simulink subsystem "Ultrasonic_Motor_Head"  (R2020b)
settings: Solver=VariableStepAuto  StartTime=0.0  StopTime=10.0  RelTol=1e-3
libraries: simulink_extras x1
settings Model: Creator=rthom  LastModifiedBy=david

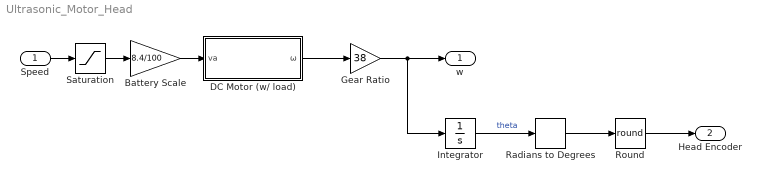
== system Ultrasonic_Motor_Head ==
  Speed : Inport
  Battery Scale : Gain  Gain=8.4/100
  DC Motor (w/ load) : Subsystem
  Gear Ratio : Gain  Gain=38
  Integrator : Integrator
  Radians to Degrees : simulink_extras/Transformations/Radians to Degrees
  Round : Rounding  Operator=round
  Saturation : Saturate  UpperLimit=100  LowerLimit=-100
  w : Outport
  Head Encoder : Outport  Port=2
  wires:
  Battery Scale/1 -> DC Motor (w/ load)/1(va)
  Round/1 -> Head Encoder/1
  Radians to Degrees/1 -> Round/1
  Integrator/1 -> Radians to Degrees/1  "theta"
  Saturation/1 -> Battery Scale/1
  Speed/1 -> Saturation/1
  Gear Ratio/1 -> Integrator/1, w/1
  DC Motor (w/ load)/1(ω) -> Gear Ratio/1

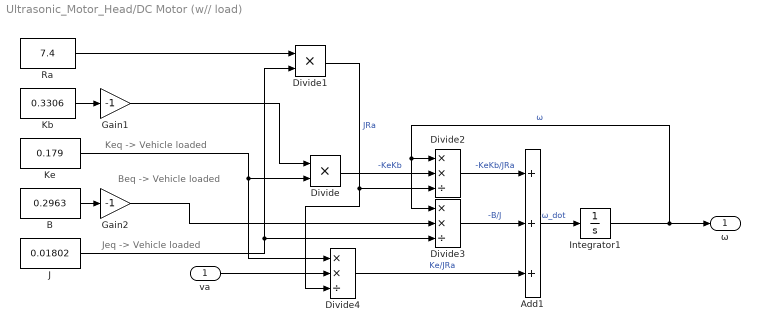
== system Ultrasonic_Motor_Head/DC Motor (w// load) ==
  note: Keq -> Vehicle loaded
  note: Jeq -> Vehicle loaded
  note: Beq -> Vehicle loaded
  va : Inport
  Add1 : Sum  Inputs=+++
  B : Constant  Value=0.2963
  Divide : Product  Inputs=**
  Divide1 : Product  Inputs=**
  Divide2 : Product  Inputs=**/
  Divide3 : Product  Inputs=**/
  Divide4 : Product  Inputs=**/
  Gain1 : Gain  Gain=-1
  Gain2 : Gain  Gain=-1
  Integrator1 : Integrator
  J : Constant  Value=0.01802
  Kb : Constant  Value=0.3306
  Ke : Constant  Value=0.179
  Ra : Constant  Value=7.4
  ω : Outport
  wires:
  Divide3/1 -> Add1/2  "-B/J"
  Add1/1 -> Integrator1/1  "ω_dot"
  J/1 -> Divide3/3, Divide1/2
  va/1 -> Divide4/2
  Ke/1 -> Divide/2, Divide4/1
  Ra/1 -> Divide1/1
  Kb/1 -> Gain1/1
  Integrator1/1 -> ω/1, Divide2/1, Divide3/1  "ω"
  Divide2/1 -> Add1/1  "-KeKb/JRa"
  Gain1/1 -> Divide/1
  Divide/1 -> Divide2/2  "-KeKb"
  Gain2/1 -> Divide3/2
  B/1 -> Gain2/1
  Divide1/1 -> Divide4/3, Divide2/3  "JRa"
  Divide4/1 -> Add1/3  "Ke/JRa"
